simulink model "ex_9_1"  (Simulink 10.1)
settings: Solver=VariableStepAuto  StartTime=0.0  StopTime=1  FixedStep=0.1  RelTol=1e-3
values from neighbouring files (symbols this model uses):
  a1 = I1 + m1 * Icl^2 + Ie + me * Ice^2 + me * L1^2    (= 3.34)    [ex_9_1.m]    (also in ex_9_2.m; ex_9_3.m)
  a2 = Ie + me * Ice^2    (= 0.97)    [ex_9_1.m]    (also in ex_9_2.m; ex_9_3.m)
  a3 = me * L1 * Ice * cos(delta_e)    [ex_9_1.m]    (also in ex_9_2.m = me_hat * L1 * Ice * cos(delta_e); ex_9_3.m = me_hat * L1 * Ice * cos(delta_e))
  a4 = me * L1 * Ice * sin(delta_e)    [ex_9_1.m]    (also in ex_9_2.m = me_hat * L1 * Ice * sin(delta_e); ex_9_3.m = me_hat * L1 * Ice * sin(delta_e))
libraries: dspmtrx3 x2
settings Model: Creator=Paulo Padrao  LastModifiedBy=Paulo Padrao
settings DataIOCC: SaveFormat=Dataset
settings OptimizationCC: LifeSpan=auto
settings DebuggingCC: UnderspecifiedInitializationDetection=Simplified  MergeDetectMultiDrivingBlocksExec=error  SFUnexpectedBacktrackingDiag=error  SFNoUnconditionalDefaultTransitionDiag=error  SFExecutionAtInitializationDiag=warning
settings HardwareCC: ProdBitPerPointer=64  ProdBitPerSizeT=64  ProdBitPerPtrDiffT=64  ProdLargestAtomicFloat=Float  ProdIntDivRoundTo=Zero  ProdEndianess=LittleEndian  ProdWordSize=64  ProdHWDeviceType=Intel->x86-64 (Windows64)
settings ModelReferenceCC: PropagateSignalLabelsOutOfModel=on
settings CodeAppCC: StateflowObjectComments=off
settings GRTTargetCC: TargetLangStandard=C99 (ISO)  CombineOutputUpdateFcns=on  GRTInterface=off
settings ConfigComp: CovMetricSettings=dwe  CovHtmlReporting=off  CovSaveCumulativeToWorkspaceVar=off  CovSaveSingleToWorkspaceVar=off  CovExternalEMLEnable=on

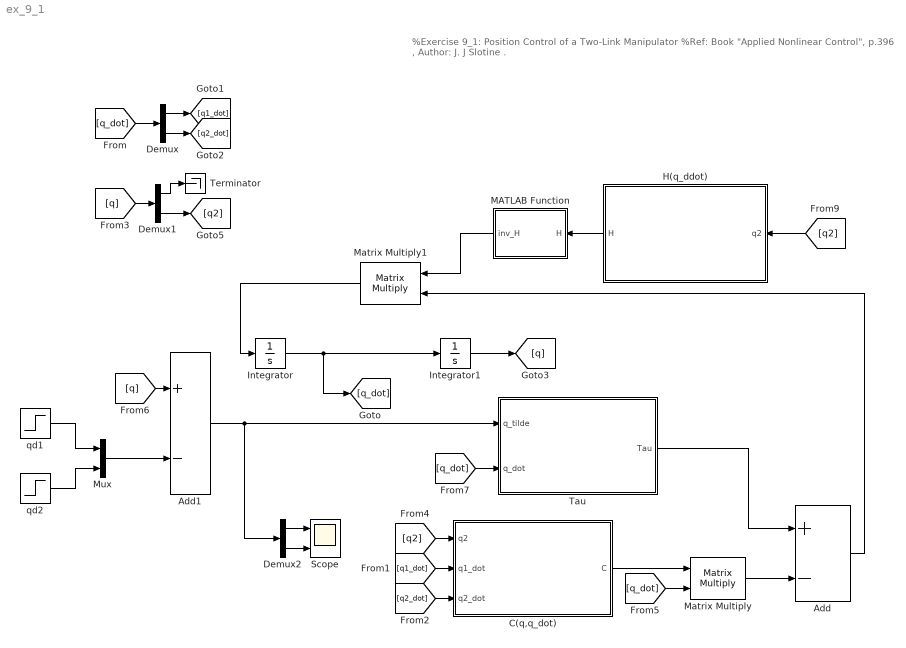
== system ex_9_1 ==
  note: %Exercise 9_1: Position Control of a Two-Link Manipulator
      | %Ref: Book "Applied Nonlinear Control", p.396 , Author: J. J Slotine .
  Add : Sum  Inputs=+-
  Add1 : Sum  Inputs=+-
  C(q,q_dot) : Subsystem
  Demux : Demux  Outputs=2
  Demux1 : Demux  Outputs=2
  Demux2 : Demux  Outputs=2
  H(q_ddot) : Subsystem
  Integrator : Integrator
  Integrator1 : Integrator
  MATLAB Function : MATLAB Function  TreatAsAtomicUnit=on
  Matrix Multiply : Product  Multiplication=Matrix(*)
  Matrix Multiply1 : Product  Multiplication=Matrix(*)
  Mux : Mux  Inputs=2
  Scope : Scope  NumInputPorts=2
  Tau : Subsystem  mask{KP=2000, KD=100}
      mask prompts: KP "Proportional Gain"; KD "Derivative Gain"
  Terminator : Terminator
  qd1 : Step  Time=0  After=60  SampleTime=0
  qd2 : Step  Time=0  After=90  SampleTime=0
  wires:
  Integrator/1 -> [q_dot], Integrator1/1
  [q_dot] -> Demux/1
  Demux/1 -> [q1_dot]
  Demux/2 -> [q2_dot]
  [q1_dot] -> C(q,q_dot)/2(q1_dot)
  [q2_dot] -> C(q,q_dot)/3(q2_dot)
  Integrator1/1 -> [q]
  [q] -> Demux1/1
  Demux1/2 -> [q2]
  [q2] -> C(q,q_dot)/1(q2)
  C(q,q_dot)/1(C) -> Matrix Multiply/1
  [q_dot] -> Matrix Multiply/2
  Tau/1(Tau) -> Add/1
  MATLAB Function/1(inv_H) -> Matrix Multiply1/1
  H(q_ddot)/1(H) -> MATLAB Function/1(H)
  [q2] -> H(q_ddot)/1(q2)
  qd1/1 -> Mux/1
  qd2/1 -> Mux/2
  [q] -> Add1/1
  Mux/1 -> Add1/2
  Add1/1 -> Demux2/1, Tau/1(q_tilde)
  [q_dot] -> Tau/2(q_dot)
  Demux1/1 -> Terminator/1
  Matrix Multiply/1 -> Add/2
  Matrix Multiply1/1 -> Integrator/1
  Add/1 -> Matrix Multiply1/2
  Demux2/2 -> Scope/2
  Demux2/1 -> Scope/1

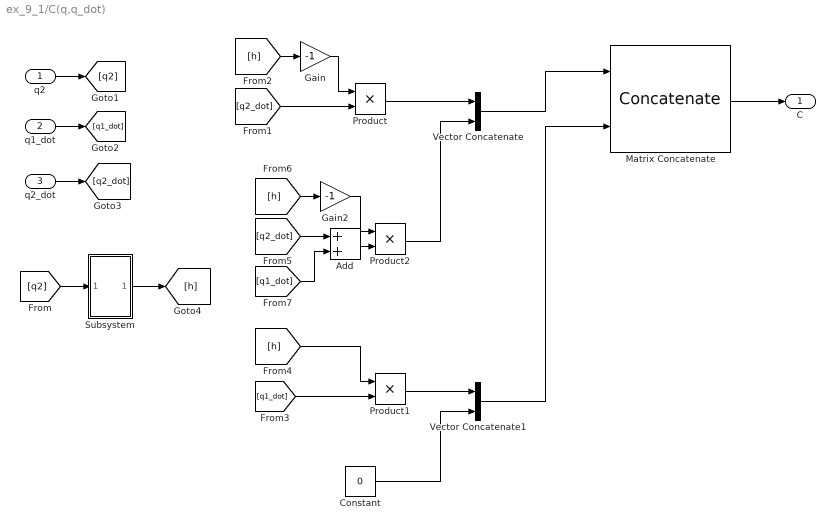
== system ex_9_1/C(q,q_dot) ==
  q2 : Inport
  q1_dot : Inport  Port=2
  q2_dot : Inport  Port=3
  Add : Sum
  Constant : Constant  Value=0
  Gain : Gain  Gain=-1
  Gain2 : Gain  Gain=-1
  Matrix Concatenate : Concatenate  Mode=Multidimensional array
  Product : Product
  Product1 : Product
  Product2 : Product
  Subsystem : Subsystem
  Vector Concatenate : Concatenate  Mode=Multidimensional array  ConcatenateDimension=2
  Vector Concatenate1 : Concatenate  Mode=Multidimensional array  ConcatenateDimension=2
  C : Outport  VectorParamsAs1DForOutWhenUnconnected=off
  wires:
  q2/1 -> [q2]
  q1_dot/1 -> [q1_dot]
  q2_dot/1 -> [q2_dot]
  [q2] -> Subsystem/1(In1)
  Subsystem/1(Out1) -> [h]
  Matrix Concatenate/1 -> C/1
  [q2_dot] -> Product/2
  [h] -> Gain/1
  Gain/1 -> Product/1
  [h] -> Product1/1
  [q1_dot] -> Product1/2
  Gain2/1 -> Product2/1
  [h] -> Gain2/1
  [q2_dot] -> Add/1
  [q1_dot] -> Add/2
  Add/1 -> Product2/2
  Product/1 -> Vector Concatenate/1
  Vector Concatenate/1 -> Matrix Concatenate/1
  Constant/1 -> Vector Concatenate1/2
  Vector Concatenate1/1 -> Matrix Concatenate/2
  Product2/1 -> Vector Concatenate/2
  Product1/1 -> Vector Concatenate1/1

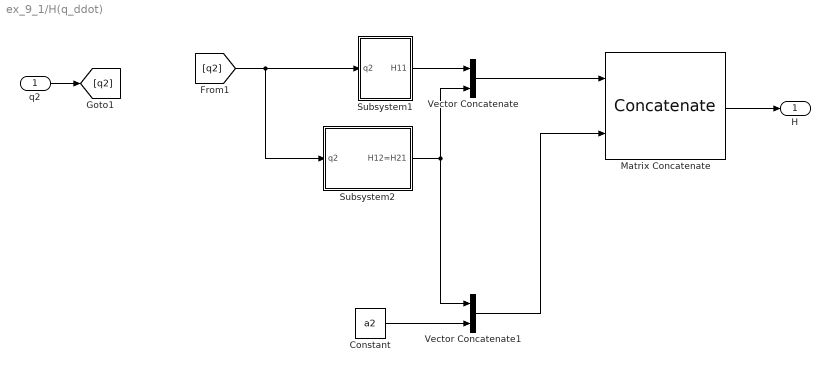
== system ex_9_1/H(q_ddot) ==
  q2 : Inport
  Constant : Constant  Value=a2
  Matrix Concatenate : Concatenate  Mode=Multidimensional array
  Subsystem1 : Subsystem
  Subsystem2 : Subsystem
  Vector Concatenate : Concatenate  Mode=Multidimensional array  ConcatenateDimension=2
  Vector Concatenate1 : Concatenate  Mode=Multidimensional array  ConcatenateDimension=2
  H : Outport  VectorParamsAs1DForOutWhenUnconnected=off
  wires:
  Vector Concatenate1/1 -> Matrix Concatenate/2
  Vector Concatenate/1 -> Matrix Concatenate/1
  Matrix Concatenate/1 -> H/1
  q2/1 -> [q2]
  Subsystem1/1("H11 ") -> Vector Concatenate/1
  [q2] -> Subsystem1/1(q2), Subsystem2/1(q2)
  Constant/1 -> Vector Concatenate1/2
  Subsystem2/1("H12=H21 ") -> Vector Concatenate1/1, Vector Concatenate/2

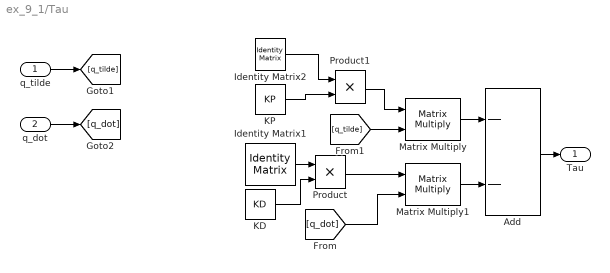
== system ex_9_1/Tau ==
  q_tilde : Inport
  q_dot : Inport  Port=2
  Add : Sum  Inputs=--
  Identity Matrix1 : dspmtrx3/Identity Matrix  Inherit=off  N=2  Ts=1  dataType=double  isSigned=on  wordLen=16  udDataType=sfix(16)  fracBitsMode=Best precision  numFracBits=15  OutDataTypeStr=double  LastOutDataTypeStr=double
  Identity Matrix2 : dspmtrx3/Identity Matrix  Inherit=off  N=2  Ts=1  dataType=double  isSigned=on  wordLen=16  udDataType=sfix(16)  fracBitsMode=Best precision  numFracBits=15  OutDataTypeStr=double  LastOutDataTypeStr=double
  KD : Constant  Value=KD
  KP : Constant  Value=KP
  Matrix Multiply : Product  Multiplication=Matrix(*)
  Matrix Multiply1 : Product  Multiplication=Matrix(*)
  Product : Product
  Product1 : Product
  Tau : Outport  VectorParamsAs1DForOutWhenUnconnected=off
  wires:
  Add/1 -> Tau/1
  q_tilde/1 -> [q_tilde]
  q_dot/1 -> [q_dot]
  Identity Matrix1/1 -> Product/1
  KD/1 -> Product/2
  [q_tilde] -> Matrix Multiply/2
  Matrix Multiply/1 -> Add/1
  KP/1 -> Product1/2
  Identity Matrix2/1 -> Product1/1
  Product1/1 -> Matrix Multiply/1
  Product/1 -> Matrix Multiply1/1
  [q_dot] -> Matrix Multiply1/2
  Matrix Multiply1/1 -> Add/2

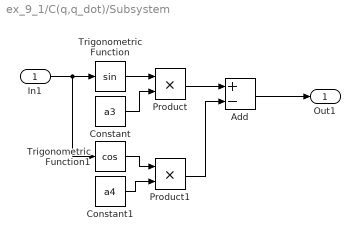
== system ex_9_1/C(q,q_dot)/Subsystem ==
  In1 : Inport
  Add : Sum  Inputs=+-
  Constant : Constant  Value=a3
  Constant1 : Constant  Value=a4
  Product : Product
  Product1 : Product
  Trigonometric Function : Trigonometry
  Trigonometric Function1 : Trigonometry  Operator=cos
  Out1 : Outport  VectorParamsAs1DForOutWhenUnconnected=off
  wires:
  Trigonometric Function1/1 -> Product1/1
  Constant/1 -> Product/2
  Product/1 -> Add/1
  Constant1/1 -> Product1/2
  In1/1 -> Trigonometric Function1/1, Trigonometric Function/1
  Trigonometric Function/1 -> Product/1
  Add/1 -> Out1/1
  Product1/1 -> Add/2

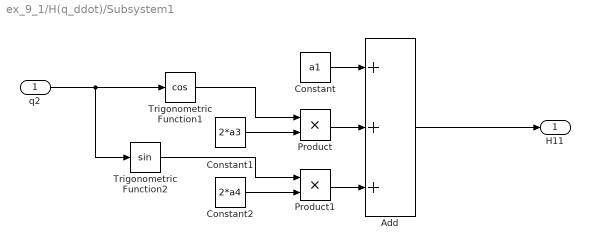
== system ex_9_1/H(q_ddot)/Subsystem1 ==
  q2 : Inport
  Add : Sum  Inputs=+++
  Constant : Constant  Value=a1
  Constant1 : Constant  Value=2*a3
  Constant2 : Constant  Value=2*a4
  Product : Product
  Product1 : Product
  Trigonometric Function1 : Trigonometry  Operator=cos
  Trigonometric Function2 : Trigonometry
  "H11 " : Outport  VectorParamsAs1DForOutWhenUnconnected=off
  wires:
  q2/1 -> Trigonometric Function1/1, Trigonometric Function2/1
  Add/1 -> "H11 "/1
  Constant/1 -> Add/1
  Product/1 -> Add/2
  Trigonometric Function1/1 -> Product/1
  Constant1/1 -> Product/2
  Constant2/1 -> Product1/2
  Trigonometric Function2/1 -> Product1/1
  Product1/1 -> Add/3

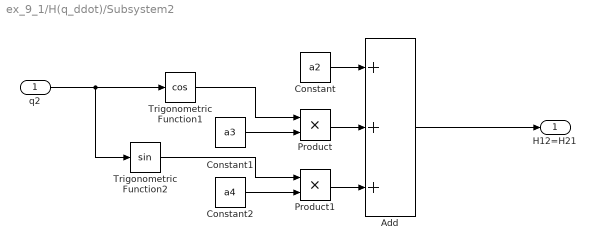
== system ex_9_1/H(q_ddot)/Subsystem2 ==
  q2 : Inport
  Add : Sum  Inputs=+++
  Constant : Constant  Value=a2
  Constant1 : Constant  Value=a3
  Constant2 : Constant  Value=a4
  Product : Product
  Product1 : Product
  Trigonometric Function1 : Trigonometry  Operator=cos
  Trigonometric Function2 : Trigonometry
  "H12=H21 " : Outport  VectorParamsAs1DForOutWhenUnconnected=off
  wires:
  Product1/1 -> Add/3
  Trigonometric Function2/1 -> Product1/1
  Constant2/1 -> Product1/2
  Constant1/1 -> Product/2
  Trigonometric Function1/1 -> Product/1
  Product/1 -> Add/2
  Constant/1 -> Add/1
  Add/1 -> "H12=H21 "/1
  q2/1 -> Trigonometric Function2/1, Trigonometric Function1/1

== matlab function MATLAB Function ==
  data: H input double; inv_H output double size=2,2
function inv_H = inv(H)

inv_H = inv(H);
